simulink model "ControlGeo"  (R2023b)
settings: Solver=ode4  StartTime=0.0  StopTime=50  FixedStep=0.001  RelTol=1e-3
settings Model: Creator=WinterFox  LastModifiedBy=WinterFox
settings DataIOCC: ReturnWorkspaceOutputs=off
settings ModelReferenceCC: ModelReferenceMinAlgLoopOccurrences=on

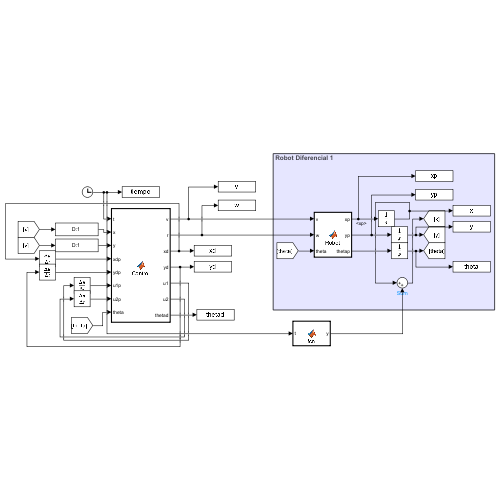
[thumbnail: Simulink's stored preview of the top-level diagram]
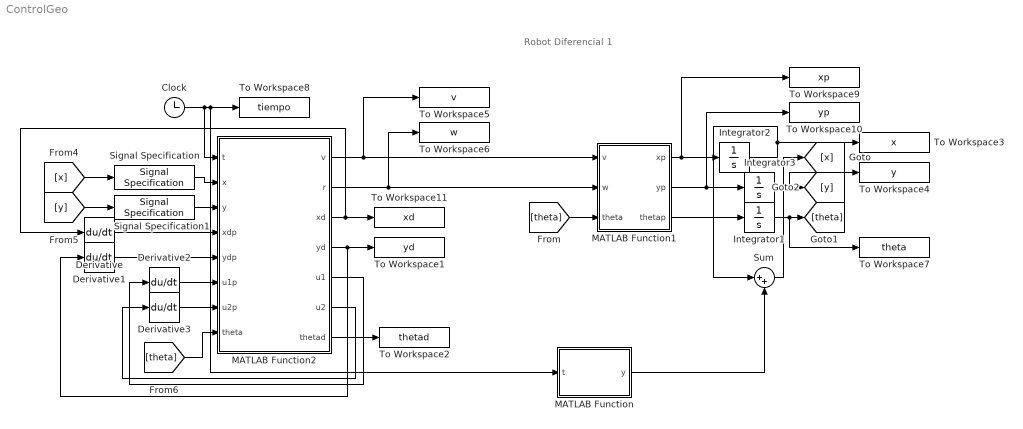
== system ControlGeo ==
  note: Robot Diferencial 1
  Clock : Clock
  Derivative{,1..3} (4 alike) : Derivative
  Integrator1 : Integrator  InitialCondition=0.1
  Integrator2 : Integrator  InitialCondition=0.1
  Integrator3 : Integrator
  MATLAB Function : MATLAB Function  TreatAsAtomicUnit=on
  MATLAB Function1 : MATLAB Function  TreatAsAtomicUnit=on
  MATLAB Function2 : MATLAB Function  TreatAsAtomicUnit=on
  Signal Specification : SignalSpecification  Dimensions=1
  Signal Specification1 : SignalSpecification  Dimensions=1
  Sum : Sum  Inputs=|++
  To Workspace1 : ToWorkspace  VariableName=yd  SampleTime=-1
  To Workspace10 : ToWorkspace  VariableName=yp  SampleTime=-1
  To Workspace11 : ToWorkspace  VariableName=xd  SampleTime=-1
  To Workspace2 : ToWorkspace  VariableName=thetad  SampleTime=-1
  To Workspace3 : ToWorkspace  VariableName=x  SampleTime=-1
  To Workspace4 : ToWorkspace  VariableName=y  SampleTime=-1
  To Workspace5 : ToWorkspace  VariableName=v  SampleTime=-1
  To Workspace6 : ToWorkspace  VariableName=w  SampleTime=-1
  To Workspace7 : ToWorkspace  VariableName=theta  SampleTime=-1
  To Workspace8 : ToWorkspace  VariableName=tiempo  SampleTime=-1
  To Workspace9 : ToWorkspace  VariableName=xp  SampleTime=-1
  wires:
  [theta] -> MATLAB Function1/3(theta)
  MATLAB Function1/1(xp) -> To Workspace9/1, Integrator2/1
  Integrator1/1 -> [theta], To Workspace7/1
  MATLAB Function1/2(yp) -> Integrator3/1, To Workspace10/1
  Integrator3/1 -> To Workspace4/1, [y]
  MATLAB Function2/1(v) -> To Workspace5/1, MATLAB Function1/1(v)
  MATLAB Function2/3(xd) -> Derivative/1, To Workspace11/1
  MATLAB Function2/4(yd) -> Derivative1/1, To Workspace1/1
  [theta] -> MATLAB Function2/8(theta)
  MATLAB Function1/3(thetap) -> Integrator1/1
  MATLAB Function2/2(r) -> To Workspace6/1, MATLAB Function1/2(w)
  [y] -> Signal Specification1/1
  [x] -> Signal Specification/1
  Clock/1 -> MATLAB Function/1(t), To Workspace8/1, MATLAB Function2/1(t)
  MATLAB Function2/7(thetad) -> To Workspace2/1
  Signal Specification/1 -> MATLAB Function2/2(x)
  Signal Specification1/1 -> MATLAB Function2/3(y)
  Derivative/1 -> MATLAB Function2/4(xdp)
  Derivative1/1 -> MATLAB Function2/5(ydp)
  Derivative2/1 -> MATLAB Function2/6(u1p)
  Derivative3/1 -> MATLAB Function2/7(u2p)
  MATLAB Function2/5(u1) -> Derivative2/1
  MATLAB Function2/6(u2) -> Derivative3/1
  MATLAB Function/1(y) -> Sum/2
  Integrator2/1 -> To Workspace3/1, Sum/1
  Sum/1 -> [x]

== matlab function ControlGeo/MATLAB Function1 ==
  data: v input size=1; w input size=1; xp output size=1; yp output size=1; theta input size=1; thetap output size=1
function [xp,yp,thetap] = Robot(v,w,theta)

xp = v*cos(theta); 
yp = v*sin(theta);
thetap = w;

== matlab function ControlGeo/MATLAB Function2 ==
  data: t input; x input; y input; xdp input; ydp input; u1p input; u2p input; v output; r output; theta input; xd output; yd output; u1 output; u2 output; thetad output
function [v,r,xd,yd,u1,u2,thetad]  = Control(t,x,y,xdp,ydp,u1p,u2p,theta)
%Parámetros de la trayectoria
%d = 0.8;
%gamma = 0.4;
a1 = 0.8;
a2 = 0.6;
p = 2*pi/50;
%Parámetros de la referencia
eps = 0.000001;
%Ganancias del controlador
k1=1;
k2=1;
k=2;
%Trayectoria lemniscata deseada
%xd = d*sqrt(2)*(sin(gamma*t/2)/(1+cos(gamma*t/2)^2));
%yd = d*sqrt(2)*(sin(gamma*t/2)*cos(gamma*t/2)/(1+cos(gamma*t/2)^2));
xd = a1*cos(p*t);
yd = a2*sin(2*p*t);
%xdp = -a1*p*sin(p*t);
%ydp = a2*2*p*cos(2*p*t);
%xdpp = -a1*p^2*cos(p*t);
%ydpp = -a2*4*p^2*sin(2*p*t);

thetad = atan2(ydp,xdp);
vd = xdp*cos(thetad)+ydp*sin(thetad);

%Rotaciones y vectores
R = [cos(theta) -sin(theta);...
     sin(theta) cos(theta)];
%Rp = [-thetap*sin(theta) -thetap*cos(theta);...
%      -thetap*cos(theta) -thetap*sin(theta)];
Rd = [cos(thetad) -sin(thetad);...
     sin(thetad) cos(thetad)];
%Rdp = [-wd*sin(thetad) -wd*cos(thetad);...
%      -wd*cos(thetad) -wd*sin(thetad)];

e1 = [1; 0];
%r = thetap;
r11 = cos(theta);
r12 = sin(theta);
%rg = [0 r;...
%      r 0];

%Sistema virtual
Xdp = vd*Rd*e1;


%Ecuaciones
KP = [k1 0;...
      0 k2];
X = [x; y];
Xd = [xd; yd];
%Xdp = [xdp; ydp];
%I = [1 0;...
%     0 1];
%Rg = Rd.'.*R;

%Errores
Xt = X-Xd;
%rt = rg-rgd;

%Control
u = -KP.*Xt+Xdp;
%v = u.'.*R.*e1;
u1 = -k1*((x-xd)+vd*r11);
u2 = -k2*((y-yd)+vd*r12);

%wd = (xdp*ydpp-ydp*xdpp)/((xdp^2+ydp^2)+eps);
wd = (u1*u2p-u2*u1p)/((norm(u)^2)+eps);

v = (u1*r11)+(u2*r12);
eomega = k*((u1*r12-u2*r11)/(norm(u)));
rd = wd;
r = rd+eomega;

== matlab function ControlGeo/MATLAB Function ==
  data: t input; y output
function y = fcn(t)

if t ==25
    y=0.2;
else
    y=0;
end
